simulink model "lavadora"  (R2021a)
settings: Solver=VariableStepAuto  StartTime=0.0  StopTime=10.0  RelTol=1e-3
libraries: fuzblock x2
settings Model: Creator=User  LastModifiedBy=User

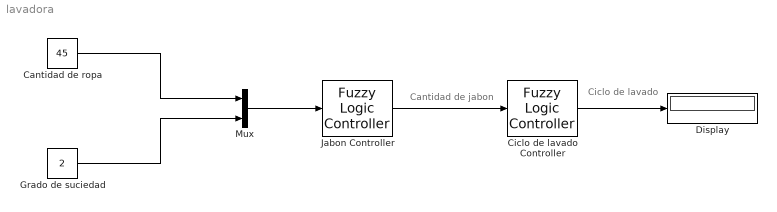
== system lavadora ==
  note: Ciclo de lavado
  note: Cantidad de jabon
  Cantidad de ropa : Constant  Value=45
  Ciclo de lavado Controller : fuzblock/Fuzzy Logic  Controller  FIS='jabon_ciclo.fis'  OutputSampleNumber=101  DataType=double  FuzzifiedInputs=off  RuleFiringStrengths=off  RuleOutputs=off  AggregatedOutputs=off  SimulateUsing=Interpreted execution  OutOfRangeInputValueMessage=warning  NoRuleFiredMessage=warning  EmptyOutputFuzzySetMessage=warning
  Display : Display
  Grado de suciedad : Constant  Value=2
  Jabon Controller : fuzblock/Fuzzy Logic  Controller  FIS='ropa_suciedad_jabon.fis'  OutputSampleNumber=101  DataType=double  FuzzifiedInputs=off  RuleFiringStrengths=off  RuleOutputs=off  AggregatedOutputs=off  SimulateUsing=Interpreted execution  OutOfRangeInputValueMessage=warning  NoRuleFiredMessage=warning  EmptyOutputFuzzySetMessage=warning
  Mux : Mux  Inputs=2
  wires:
  Jabon Controller/1 -> Ciclo de lavado Controller/1
  Cantidad de ropa/1 -> Mux/1
  Mux/1 -> Jabon Controller/1
  Grado de suciedad/1 -> Mux/2
  Ciclo de lavado Controller/1 -> Display/1
